simulink model "Observer_sfun"  (R2020b)
settings: Solver=VariableStepAuto  StartTime=0.0  StopTime=30  RelTol=1e-3
settings Model: Creator=zhiyao  LastModifiedBy=zhiyao

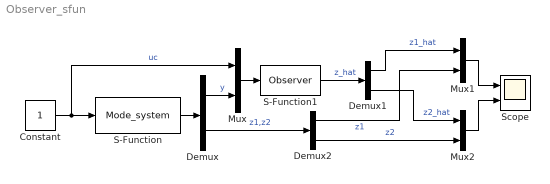
== system Observer_sfun ==
  Constant : Constant
  Demux : Demux  Outputs=2
  Demux1 : Demux  Outputs=2
  Demux2 : Demux  Outputs=2
  Mux : Mux  Inputs=2
  Mux1 : Mux  Inputs=2
  Mux2 : Mux  Inputs=2
  S-Function : S-Function  FunctionName=Mode_system  SFunctionDeploymentMode=off  EnableBusSupport=off
  S-Function1 : S-Function  FunctionName=Observer  SFunctionDeploymentMode=off  EnableBusSupport=off
  Scope : Scope  NumInputPorts=2
  wires:
  Constant/1 -> Mux/1, S-Function/1  "uc"
  S-Function/1 -> Demux/1
  Mux/1 -> S-Function1/1
  Demux/1 -> Mux/2  "y"
  S-Function1/1 -> Demux1/1  "z_hat"
  Demux1/1 -> Mux1/1  "z1_hat"
  Demux/2 -> Demux2/1  "z1,z2"
  Demux2/2 -> Mux2/2  "z2"
  Demux1/2 -> Mux2/1  "z2_hat"
  Demux2/1 -> Mux1/2  "z1"
  Mux1/1 -> Scope/1
  Mux2/1 -> Scope/2
